simulink model "PlutoSim"  (R2024b)
settings: Solver=VariableStepAuto  StartTime=0.0  StopTime=1  RelTol=1e-3
undefined symbols (not defined in the file): Fs, ip, usb
libraries: commutil2 x3, commdigbbndpm3 x3, plutoradiolib x2, commseqgen3 x2, commsync2 x2, dspstat3 x2, commfilt2 x2, commrfcorlib x1, commsink2 x1, commrandsrc3 x1
settings Model: Creator=skaug  LastModifiedBy=skaug

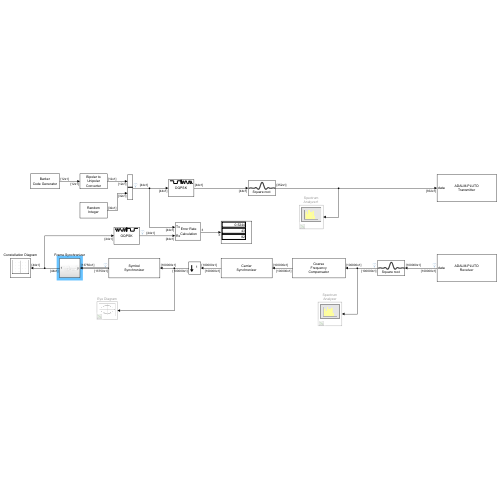
[thumbnail: Simulink's stored preview of the top-level diagram]
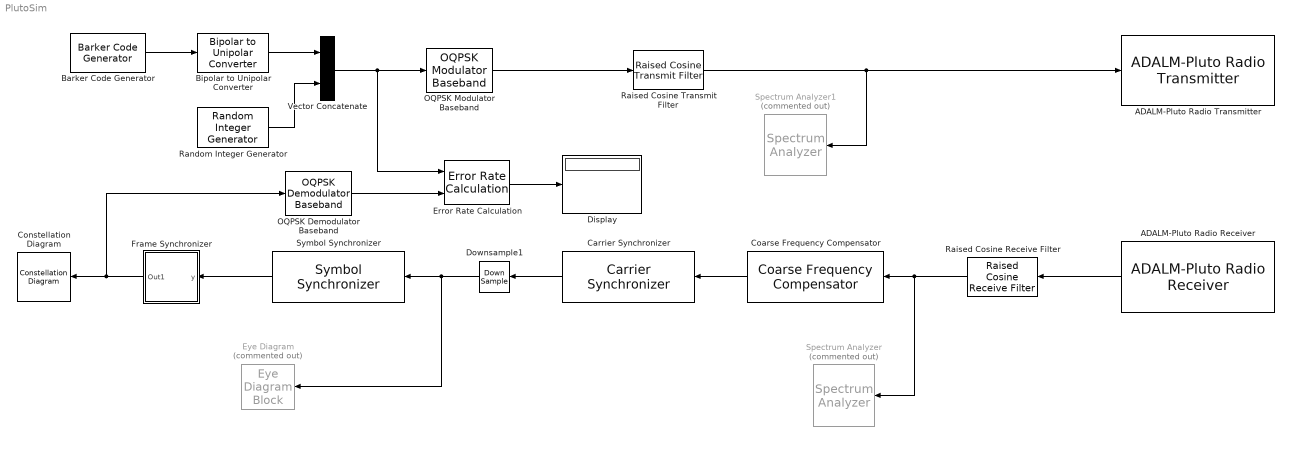
== system PlutoSim ==
  ADALM-Pluto Radio Receiver : plutoradiolib/ADALM-Pluto Radio Receiver  RadioID=usb:0  uri=ip:10.0.0.200  CenterFrequencySource=Dialog  CenterFrequency=0.8e9  GainSource=AGC Slow Attack  GainSourceBlock=AGC Slow Attack  Gain=10  ChannelMapping=1  BasebandSampleRate=1e5  OutputDataType=double  SamplesPerFrame=1e5  OverflowOutputPort=off  EnableBurstMode=off  NumFramesInBurst=1  ShowAdvancedProperties=off  UseCustomFilter=off  filtPathRates=[737280000 11520000 3840000 1920000 960000 240000]  filtCoefficients=[-192 82 85 -215 228 -102 -110 290 -318 145 160 -426 471 -215 -238 633 -697 318 349 -923 1009 -457 -498 1309 -1423 640 693 -1812 1959 -876 -945 2458 -2647 1180 1268 -3290 3534 -1572 -1688 4375 -4698 2091 2247 -5836 6284 -2807 -3031 7918 -8588 3870 4225 -11182 12324 -5662 -6330 17255 -19735 9507 11312 -33568 43355 -25227 -42139 305542 305542 -42139 -25227 43355 -33568 11312 9507 -19735 17255 -6330 -5662 12324 -11182 4225 3870 -8588 7918 -3031 -2807 6284 -5836 2247 2091 -4698 4375 -1688 -1572 3534 -3290 1268 1180 -2647 2458 -945 -876 1959 -1812 693 640 -1423 1309 -498 -457 1009 -923 349 318 -697 633 -238 -215 471 -426 160 145 -318 290 -110 -102 228 -215 85 82 -192]  filtCoefficientSize=128  filtDecimInterpFactor=4  filtGain=-12  filtRFBandwidth=18000000  filterConfigStruct=struct()  EnableQuadratureCorrection=on  EnableRFDCCorrection=on  EnableBasebandDCCorrection=on  FrequencyCorrection=0  OverrideSampleTime=off  SampleTime=0.02  DataTimeout=Inf  ENSMPinControlMode=None  BISTLoopbackMode=Disabled  BISTToneInject=Disabled  BISTSignalGen=PRBS  BISTToneFreq=Fs/32  BISTToneLevel=0
  ADALM-Pluto Radio Transmitter : plutoradiolib/ADALM-Pluto Radio Transmitter  RadioID=usb:0  uri=ip:10.0.0.200  CenterFrequencySource=Dialog  CenterFrequency=0.8e9  GainSource=Dialog  Gain=0  ChannelMapping=1  BasebandSampleRate=1e5  UnderflowOutputPort=off  ShowAdvancedProperties=off  UseCustomFilter=off  filtPathRates=[737280000 11520000 3840000 1920000 960000 240000]  filtCoefficients=[-192 82 85 -215 228 -102 -110 290 -318 145 160 -426 471 -215 -238 633 -697 318 349 -923 1009 -457 -498 1309 -1423 640 693 -1812 1959 -876 -945 2458 -2647 1180 1268 -3290 3534 -1572 -1688 4375 -4698 2091 2247 -5836 6284 -2807 -3031 7918 -8588 3870 4225 -11182 12324 -5662 -6330 17255 -19735 9507 11312 -33568 43355 -25227 -42139 305542 305542 -42139 -25227 43355 -33568 11312 9507 -19735 17255 -6330 -5662 12324 -11182 4225 3870 -8588 7918 -3031 -2807 6284 -5836 2247 2091 -4698 4375 -1688 -1572 3534 -3290 1268 1180 -2647 2458 -945 -876 1959 -1812 693 640 -1423 1309 -498 -457 1009 -923 349 318 -697 633 -238 -215 471 -426 160 145 -318 290 -110 -102 228 -215 85 82 -192]  filtCoefficientSize=128  filtDecimInterpFactor=4  filtGain=-12  filtRFBandwidth=18000000  filterConfigStruct=struct()  DataSourceSelect=Input Port  DDSTone1Freq=5e3  DDSTone2Freq=10e3  DDSTone1Scale=0.5  DDSTone2Scale=0.25  DataTimeout=Inf  FrequencyCorrection=0  ENSMPinControlMode=None  BISTLoopbackMode=Disabled  BISTToneInject=Disabled  BISTSignalGen=PRBS  BISTToneFreq=Fs/32  BISTToneLevel=0
  Barker Code Generator : commseqgen3/Barker Code Generator  Length=7  LengthSimulink=13  SampleTime=-1  SamplesPerFrame=12  OutputDataType=double  SimulateUsing=Code generation
  Bipolar to Unipolar Converter : commutil2/Bipolar to Unipolar Converter  M=2  polarity=Positive  dataType=Inherit via internal rule
  Carrier Synchronizer : commsync2/Carrier Synchronizer  Modulation=OQPSK  ModulationPhaseOffset=Auto  CustomPhaseOffset=0  SamplesPerSymbol=8  DampingFactor=0.707  NormalizedLoopBandwidth=0.01  EstimatedPhaseErrorOutputPort=off  SimulateUsing=Code generation
  Coarse Frequency Compensator : commrfcorlib/Coarse Frequency Compensator  Modulation=OQPSK  Algorithm=FFT-based  FrequencyResolution=100  MaximumFrequencyOffset=5e3  SamplesPerSymbol=8  EstimatedFreqOffsetPort=off  SimulateUsing=Code generation
      settings: LibrarySourceBlock=|
      | commsync2/Coarse Frequency
      | Compensator
  Constellation Diagram : ConstellationDiagram  WindowPosition=[452.000000,158.000000,1169.000000,730.000000,]  ScopeFrameLocation=window  ReferenceConstellation="[0.7071+0.7071i          -0.7071+0.7071i          -0.7071-0.7071i            0.707-0.7071i]"  ShowLegend=on
  Display : Display
  Downsample1 : DownSample  N=1
  Error Rate Calculation : commsink2/Error Rate Calculation  N=6  st_delay=0  cp_mode=Entire frame  subframe=[]  PMode=Port  WsName=ErrorVec  RsMode2=off  stop=off  numErr=100  maxBits=1e6
  Eye Diagram : EyeDiagramBlock  Commented=on  WindowPosition=[962.000000,169.000000,817.000000,543.000000,]  ScopeFrameLocation=window
  Frame Synchronizer : Subsystem
  OQPSK Demodulator Baseband : commdigbbndpm3/OQPSK Demodulator Baseband  OutType=Bit  Ph=pi/4  Mapping=Gray  pulseShape=Half sine  num=[0.7071, 0.7071]  rolloff=0.2  filterSpan=10  sps=2  RateOptions=Enforce single-rate processing  outDtype2=double
  OQPSK Modulator Baseband : commdigbbndpm3/OQPSK Modulator Baseband  VariantControl=strcmp(pulseShape, 'Custom') && isequal(denom, 1)  InType=Bit  Mapping=Gray  Ph=pi/4  pulseShape=Half sine  num=[0.7071, 0.7071]  denom=[1]  rolloff=0.2  filterSpan=10  sps=2  RateOptions=Enforce single-rate processing  outDtype=double  isIIR=off
  Raised Cosine Receive Filter : commfilt2/Raised Cosine Receive Filter  filtType=Square root  R=0.35  filtSpan=4  N=8  downFactor=1  downOffset=0  filterGain=1  InputProcessing=Columns as channels (frame based)  RateOptions=Enforce single-rate processing  framing=Mute  checkCoeff=off  variableName=rcRxFilt  currentFiltSpan=10  D=5  inputOffset=0  sampMode=Mute  saveAsFlag=0  rateMode=Downsampling  checkGain=Normalized  launchFVT=on  roundingMode=Floor  overflowMode=off  coeffDataTypeStr=Inherit: Same word length as input  coeffMin=[]  coeffMax=[]  coeffLastDataTypeStr=Inherit: Same word length as input  accumDataTypeStr=Inherit: Same as product output  accumLastDataTypeStr=Inherit: Same as product output  outputDataTypeStr=Inherit: Same as accumulator  outputMin=[]  outputMax=[]  outputLastDataTypeStr=Inherit: Same as accumulator
      settings: LibrarySourceBlock=|
      | commhdlfilt/Raised Cosine
      | Receive Filter
  Raised Cosine Transmit Filter : commfilt2/Raised Cosine Transmit Filter  filtType=Square root  R=0.35  filtSpan=4  N=8  filterGain=1  InputProcessing=Columns as channels (frame based)  RateOptions=Enforce single-rate processing  framing=Mute  checkCoeff=off  variableName=rcTxFilt  checkGain=Normalized  sampMode=Mute  saveAsFlag=0  currentFiltSpan=10  D=5  launchFVT=on  roundingMode=Floor  overflowMode=off  coeffDataTypeStr=Inherit: Same word length as input  coeffMin=[]  coeffMax=[]  coeffLastDataTypeStr=Inherit: Same word length as input  outputDataTypeStr=Inherit: Same as accumulator  outputMin=[]  outputMax=[]  outputLastDataTypeStr=Inherit: Same as accumulator
      settings: LibrarySourceBlock=|
      | commhdlfilt/Raised Cosine
      | Transmit Filter
  Random Integer Generator : commrandsrc3/Random Integer Generator  SetSize=2  SeedSource=Auto  Seed=0  SampleTime=-1  SamplesPerFrame=32  OutputDataType=double  SimulateUsing=Interpreted execution
  Spectrum Analyzer : SpectrumAnalyzer  Tag=simrfV2util1/Spectrum Analyzer  Commented=on  WindowPosition=[368.000000,488.000000,1331.000000,721.000000,]  ScopeFrameLocation=window  Method=Welch  AveragingMethod=Exponential  YLimits=[-80.22972228568331,13.852155026833934]  SelectedToolstripTab=spectrumAnalyzerToolstrip.channelMeasurementsTab  AllowFFTLengthLessThanSamplesPerUpdate=on
  Spectrum Analyzer1 : SpectrumAnalyzer  Tag=simrfV2util1/Spectrum Analyzer  Commented=on  WindowPosition=[386.000000,437.000000,1331.000000,721.000000,]  ScopeFrameLocation=window  Method=Welch  AveragingMethod=Exponential  YLimits=[-112.75907922079537,49.472186202190024]  SelectedToolstripTab=spectrumAnalyzerToolstrip.channelMeasurementsTab  AllowFFTLengthLessThanSamplesPerUpdate=on
  Symbol Synchronizer : commsync2/Symbol Synchronizer  Modulation=OQPSK  TimingErrorDetector=Gardner (non-data-aided)  SamplesPerSymbol=8  DampingFactor=1  NormalizedLoopBandwidth=0.01  DetectorGain=5.4  TimingErrorOutputPort=off  SimulateUsing=Code generation
  Vector Concatenate : Concatenate
  wires:
  Raised Cosine Receive Filter/1 -> Spectrum Analyzer/1, Coarse Frequency Compensator/1
  OQPSK Modulator Baseband/1 -> Raised Cosine Transmit Filter/1
  Barker Code Generator/1 -> Bipolar to Unipolar Converter/1
  Bipolar to Unipolar Converter/1 -> Vector Concatenate/1
  Random Integer Generator/1 -> Vector Concatenate/2
  Vector Concatenate/1 -> Error Rate Calculation/1, OQPSK Modulator Baseband/1
  Coarse Frequency Compensator/1 -> Carrier Synchronizer/1
  Carrier Synchronizer/1 -> Downsample1/1
  Raised Cosine Transmit Filter/1 -> Spectrum Analyzer1/1, ADALM-Pluto Radio Transmitter/1
  Downsample1/1 -> Eye Diagram/1, Symbol Synchronizer/1
  Frame Synchronizer/1(Out1) -> OQPSK Demodulator Baseband/1, Constellation Diagram/1
  Symbol Synchronizer/1 -> Frame Synchronizer/1(y)
  ADALM-Pluto Radio Receiver/1 -> Raised Cosine Receive Filter/1
  OQPSK Demodulator Baseband/1 -> Error Rate Calculation/2
  Error Rate Calculation/1 -> Display/1

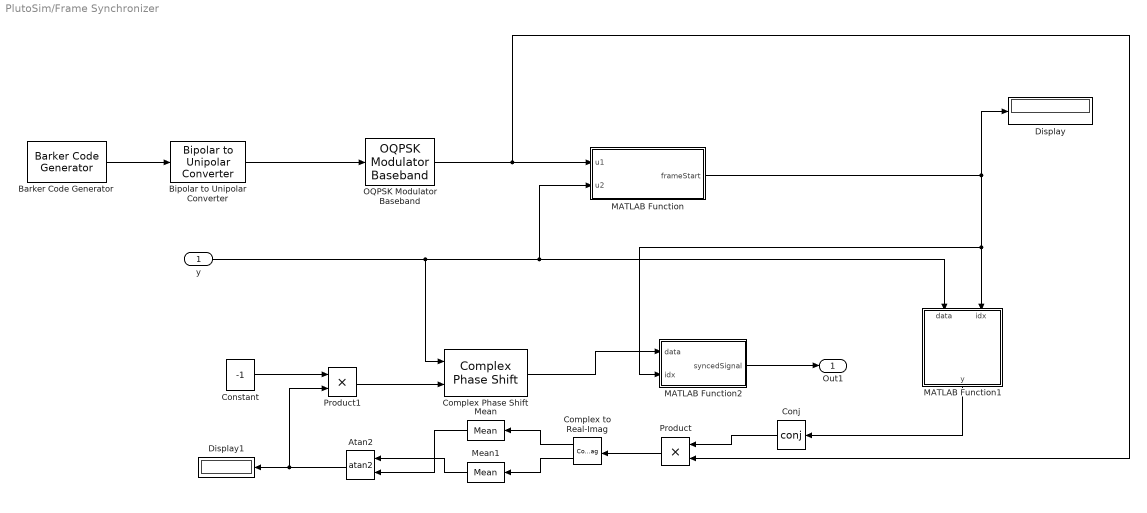
== system PlutoSim/Frame Synchronizer ==
  y : Inport
  Atan2 : Trigonometry  Operator=atan2
  Barker Code Generator : commseqgen3/Barker Code Generator  Length=7  LengthSimulink=13  SampleTime=-1  SamplesPerFrame=12  OutputDataType=double  SimulateUsing=Code generation
  Bipolar to Unipolar Converter : commutil2/Bipolar to Unipolar Converter  M=2  polarity=Positive  dataType=Inherit via internal rule
  Complex Phase Shift : commutil2/Complex Phase Shift
  Complex to Real-Imag : ComplexToRealImag
  Conj : Math  Operator=conj
  Constant : Constant  Value=-1  VectorParams1D=off  SampleTime=-1
  Display : Display
  Display1 : Display
  MATLAB Function : MATLAB Function  TreatAsAtomicUnit=on
  MATLAB Function1 : MATLAB Function  TreatAsAtomicUnit=on
  MATLAB Function2 : MATLAB Function  TreatAsAtomicUnit=on
  Mean : dspstat3/Mean  run=off  InputProcessing=Columns as channels (frame based)  reset_popup=None  directionMode=Each column  dimension=1  roiEnable=off  roiType=Rectangles  roiPortion=Entire ROI  roiOutput=Individual statistics for each ROI  roiFlag=off  roundingMode=Floor  overflowMode=off  outputDataTypeStr=Inherit: Same as accumulator  outputMin=[]  outputMax=[]  outputLastDataTypeStr=Inherit: Same as accumulator
  Mean1 : dspstat3/Mean  run=off  InputProcessing=Columns as channels (frame based)  reset_popup=None  directionMode=Each column  dimension=1  roiEnable=off  roiType=Rectangles  roiPortion=Entire ROI  roiOutput=Individual statistics for each ROI  roiFlag=off  roundingMode=Floor  overflowMode=off  outputDataTypeStr=Inherit: Same as accumulator  outputMin=[]  outputMax=[]  outputLastDataTypeStr=Inherit: Same as accumulator
  OQPSK Modulator Baseband : commdigbbndpm3/OQPSK Modulator Baseband  VariantControl=strcmp(pulseShape, 'Custom') && isequal(denom, 1)  InType=Bit  Mapping=Gray  Ph=pi/4  pulseShape=Half sine  num=[0.7071, 0.7071]  denom=[1]  rolloff=0.2  filterSpan=10  sps=2  RateOptions=Enforce single-rate processing  outDtype=double  isIIR=off
  Product : Product
  Product1 : Product
  Out1 : Outport
  wires:
  OQPSK Modulator Baseband/1 -> Product/2, MATLAB Function/1(u1)
  y/1 -> MATLAB Function1/1(data), MATLAB Function/2(u2), Complex Phase Shift/1
  Barker Code Generator/1 -> Bipolar to Unipolar Converter/1
  Bipolar to Unipolar Converter/1 -> OQPSK Modulator Baseband/1
  MATLAB Function/1(frameStart) -> MATLAB Function2/2(idx), MATLAB Function1/2(idx), Display/1
  Conj/1 -> Product/1
  Product/1 -> Complex to Real-Imag/1
  Complex to Real-Imag/2 -> Mean1/1
  Complex to Real-Imag/1 -> Mean/1
  Mean1/1 -> Atan2/1
  Mean/1 -> Atan2/2
  Atan2/1 -> Product1/2, Display1/1
  Complex Phase Shift/1 -> MATLAB Function2/1(data)
  Product1/1 -> Complex Phase Shift/2
  Constant/1 -> Product1/1
  MATLAB Function1/1(y) -> Conj/1
  MATLAB Function2/1(syncedSignal) -> Out1/1

== matlab function PlutoSim/Frame Synchronizer/MATLAB Function ==
  data: u1 input; frameStart output; u2 input
function frameStart = findFrameStart(u1, u2)

    [corr, lags] = xcorr(u2, u1);
    [~, idx] = max(abs(corr));
    
    frameStart = lags(idx) + 1;

== matlab function PlutoSim/Frame Synchronizer/MATLAB Function2 ==
  data: data input; syncedSignal output; idx input
function syncedSignal = frameSync(data,idx)
syncedSignal=data(idx:idx+43); % len(frame) - 1

== matlab function PlutoSim/Frame Synchronizer/MATLAB Function1 ==
  data: data input; y output; idx input
function y = rxTrainingSignal(data,idx)
y=data(idx:idx+11);
